simulink model "Pitch1doF"  (R2019b)
settings: Solver=VariableStepAuto  StartTime=0.0  StopTime=10.0  RelTol=1e-3
undefined symbols (not defined in the file): Dm, Dt, g, Jp, K_pitch, Mb
libraries: cstblocks x2
settings Model: Creator=lbend  LastModifiedBy=lbend

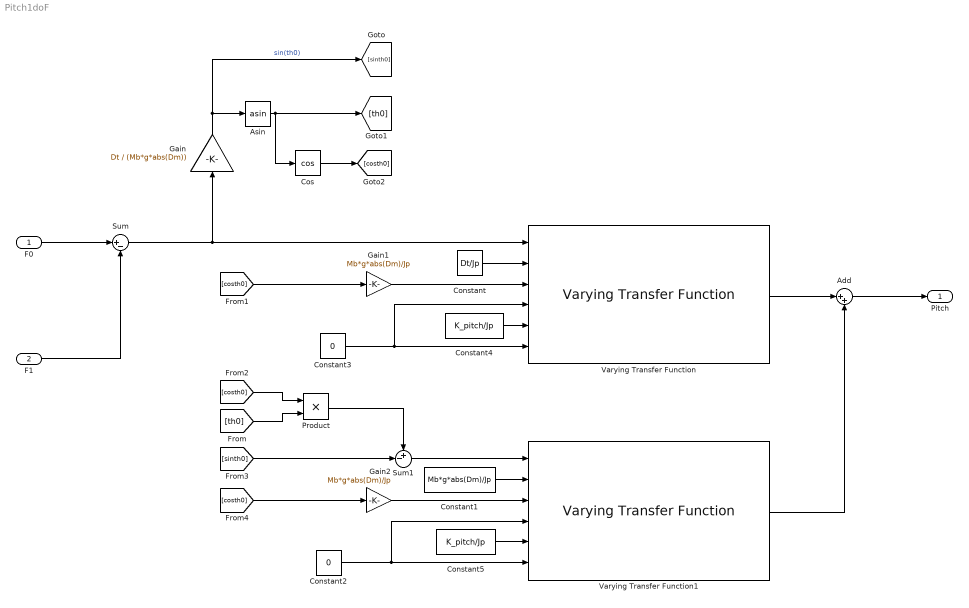
== system Pitch1doF ==
  F0 : Inport
  F1 : Inport  Port=2
  Add : Sum  Inputs=|++
  Asin : Trigonometry  Operator=asin
  Constant : Constant  Value=Dt/Jp
  Constant1 : Constant  Value=Mb*g*abs(Dm)/Jp
  Constant2 : Constant  Value=0
  Constant3 : Constant  Value=0
  Constant4 : Constant  Value=K_pitch/Jp
  Constant5 : Constant  Value=K_pitch/Jp
  Cos : Trigonometry  Operator=cos
  Gain : Gain  Gain=Dt / (Mb*g*abs(Dm))
  Gain1 : Gain  Gain=Mb*g*abs(Dm)/Jp
  Gain2 : Gain  Gain=Mb*g*abs(Dm)/Jp
  Product : Product
  Sum : Sum  Inputs=|+-
  Sum1 : Sum  Inputs=+-|
  Varying Transfer Function : cstblocks/Linear Parameter Varying/Varying Transfer Function  N=2
      settings: SourceProductName=Control System Toolbox
  Varying Transfer Function1 : cstblocks/Linear Parameter Varying/Varying Transfer Function  N=2
      settings: SourceProductName=Control System Toolbox
  Pitch : Outport
  wires:
  [th0] -> Product/2
  [costh0] -> Gain1/1
  [costh0] -> Product/1
  [sinth0] -> Sum1/2
  Gain2/1 -> Varying Transfer Function1/3
  Product/1 -> Sum1/1
  Varying Transfer Function1/1 -> Add/2
  Constant/1 -> Varying Transfer Function/2
  Gain/1 -> Asin/1, [sinth0]  "sin(th0)"
  Sum/1 -> Gain/1, Varying Transfer Function/1
  Gain1/1 -> Varying Transfer Function/3
  Asin/1 -> [th0], Cos/1
  Sum1/1 -> Varying Transfer Function1/1
  Constant2/1 -> Varying Transfer Function1/6, Varying Transfer Function1/4
  Varying Transfer Function/1 -> Add/1
  Constant1/1 -> Varying Transfer Function1/2
  Constant3/1 -> Varying Transfer Function/6, Varying Transfer Function/4
  Constant4/1 -> Varying Transfer Function/5
  Cos/1 -> [costh0]
  F1/1 -> Sum/2
  [costh0] -> Gain2/1
  F0/1 -> Sum/1
  Constant5/1 -> Varying Transfer Function1/5
  Add/1 -> Pitch/1
